simulink model "cdnlink_lb_wide_15a"  (Simulink 8.5)
settings: Solver=ode45  StartTime=0.0  StopTime=10.0  RelTol=1e-3
undefined symbols (not defined in the file): des, gcbh
(part 1 of 3)
settings Model: Creator=erwin2h  LastModifiedBy=erwin2h
settings DataIOCC: SignalLoggingSaveFormat=Dataset
settings OptimizationCC: ExpressionDepthLimit=128
settings DebuggingCC: UnderspecifiedInitializationDetection=Simplified  MergeDetectMultiDrivingBlocksExec=error  FcnCallInpInsideContextMsg=EnableAllAsError  StateNameClashWarn=none
settings GRTTargetCC: CombineOutputUpdateFcns=on  GRTInterface=off

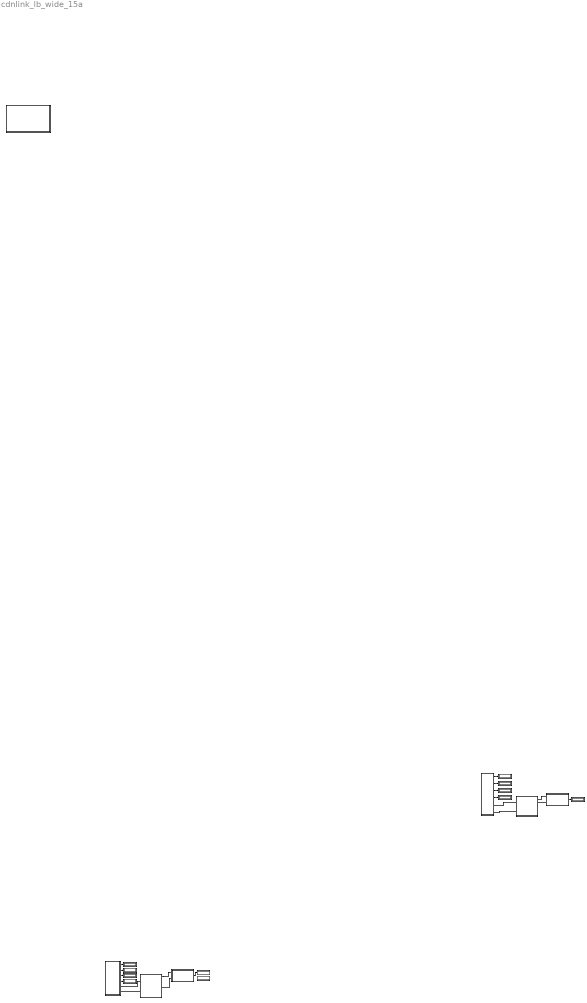
== system cdnlink_lb_wide_15a ==
  note: CDNLink
  note: Load Balancing Simulator
  note: Erwin Harahap
      | (R) 2015. Hiroaki Nishi Laboratory
      | Keio University, Yokohama.
      | Japan
  note: Last update: Sept 2015
  note: Fukuoka
  note: 1
  note: Kurashiki
  note: 3
  C1 : Subsystem
      mask Display: disp('Client 1');
  C3 : Subsystem
      mask Display: disp('Client\nv.2.0');
  Display{1..5,53,83..86,89} (11 alike) : Display
  Instrumentation : Subsystem
      mask Display: disp('Instrumentation')
  R1 : Subsystem
      mask Display: disp('Router 1');
  R3 : Subsystem
  S1 : Subsystem
      mask Display: disp('Surrogate Server 1');
  S3 : Subsystem
      mask Display: disp('Surrogate Server 1');
  wires:
  C1/1(Req sent) -> Display83/1
  C1/2(DNS sent) -> Display84/1
  C1/3(Req drop) -> Display85/1
  C1/4(DNS drop) -> Display86/1
  S1/1(Out1) -> Display89/1
  ? -> Display53/1
  C3/1(Req sent) -> Display1/1
  C3/2(DNS sent) -> Display2/1
  C3/3(Req drop) -> Display3/1
  C3/4(DNS drop) -> Display4/1
  S3/1(Out1) -> Display5/1
  connections:
  R1/RConn1 -- S1/LConn1
  S1/LConn2 -- R1/RConn5
  R1/LConn2 -- C1/RConn2
  R1/LConn1 -- C1/RConn1
  R3/LConn1 -- C3/RConn1
  R3/LConn2 -- C3/RConn2
  S3/LConn1 -- R3/RConn1
  S3/LConn2 -- R3/RConn2

== system cdnlink_lb_wide_15a/C1 ==
  note: CDNLink
  note: Client 1
  note: Erwin Harahap
      | (c) 2015. Hiroaki Nishi Laboratory
      | Keio University
      | Japan
  note: Ver. 2.0
  Packet Request Generator : Subsystem
      mask Display: disp('Packet \nGenerator')
  Processing Module1 : Subsystem
      mask Display: disp('Processing\nModule')
  Sink : Subsystem
      mask Display: disp('Sink')
  to router : PMIOPort  Port=1  Side=Right
  from Router : PMIOPort  Port=2  Side=Right
  Req sent : Outport
  DNS sent : Outport  Port=2
  Req drop : Outport  Port=3
  DNS drop : Outport  Port=4
  wires:
  Packet Request Generator/1(Out1) -> Req sent/1
  Packet Request Generator/2(Out2) -> DNS sent/1
  Sink/1(Out1) -> Req drop/1
  Sink/2(Out2) -> DNS drop/1
  connections:
  Processing Module1/LConn1 -- Packet Request Generator/RConn1
  Processing Module1/LConn2 -- from Router/RConn1
  Processing Module1/RConn1 -- to router/RConn1
  Processing Module1/RConn2 -- Sink/LConn1

== system cdnlink_lb_wide_15a/C3 ==
  note: Standard:
      | Arrival rate : 20 pkt/second = 1/20 = 0.05 sec/packet
      | Client service rate = 5 Mbps = 5*10^6 bps = 5*10^3/12 = 0.42*10^3 = 420 packet/second = 0.0024 s/packet = 2.4 ms/packet
      | Server service rate 10 Mbps = 10*10^6 bps = 10*10^3/12 = 0.83*10^3 = 830 packet/second = 0.0012 s/packet
      | SoR service rate : 10 Mbps
      | One packet size : 1500 bytes = 12000bps
      | 1 ms/packet = 1008 packet/s
  note: CDNLink
  note: Client 3
  Packet Request Generator : Subsystem
      mask Display: disp('Packet Generator\nv.1.02')
  Processing Module1 : Subsystem
      mask Display: disp('Client Processing Module\nv.1.03')
  Sink1 : Subsystem
      mask Display: disp('Sink')
  from Router : PMIOPort  Port=1  Side=Right
  to router : PMIOPort  Port=2  Side=Right
  Req sent : Outport
  DNS sent : Outport  Port=2
  Req drop : Outport  Port=3
  DNS drop : Outport  Port=4
  wires:
  Packet Request Generator/1(Out1) -> Req sent/1
  Packet Request Generator/2(Out2) -> DNS sent/1
  Sink1/1(Out1) -> Req drop/1
  Sink1/2(Out2) -> DNS drop/1
  connections:
  Processing Module1/LConn1 -- Packet Request Generator/RConn1
  Processing Module1/LConn2 -- from Router/RConn1
  Processing Module1/RConn1 -- to router/RConn1
  Sink1/LConn1 -- Processing Module1/RConn2

== system cdnlink_lb_wide_15a/Instrumentation ==
  note: CDNLink
  note: Instrumentation & Packet Monitoring
  note: v.1.0

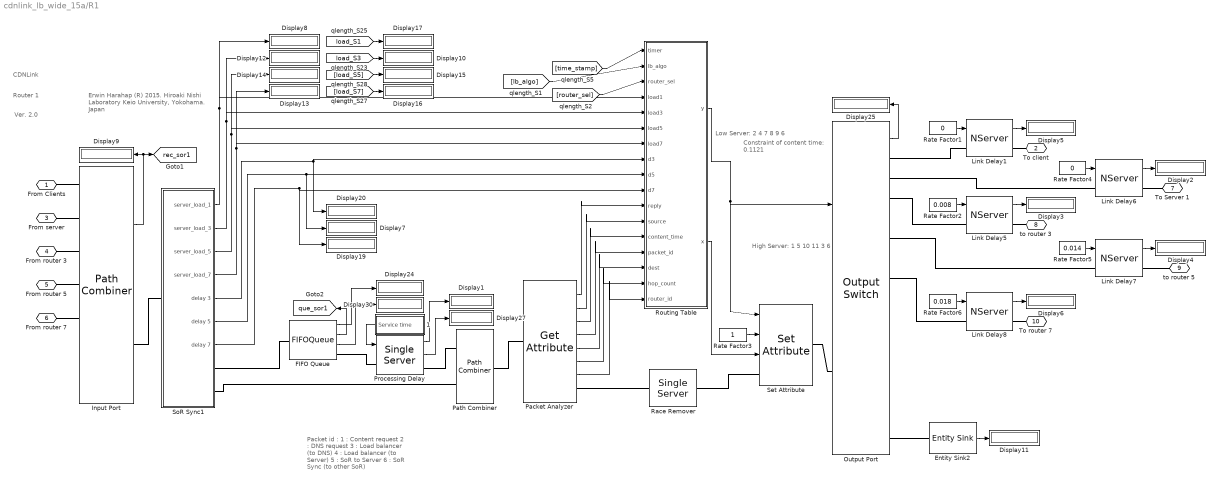
== system cdnlink_lb_wide_15a/R1 ==
  note: CDNLink
  note: Router 1
  note: High Server:
      | 1
      | 5
      | 10
      | 11
      | 3
      | 6
  note: Packet id :
      | 1 : Content request
      | 2 : DNS request
      | 3 : Load balancer (to DNS)
      | 4 : Load balancer (to Server)
      | 5 : SoR to Server
      | 6 : SoR Sync (to other SoR)
  note: Constraint of content time:
      | 0.1121
  note: Erwin Harahap
      | (R) 2015. Hiroaki Nishi Laboratory
      | Keio University, Yokohama.
      | Japan
  note: Low Server:
      | 2
      | 4
      | 7
      | 8
      | 9
      | 6
  note: Ver. 2.0
  " 1" : Subsystem
      mask Display: disp('M/M/1 Gen');
  Display{1..17,19..20,24..25,27,30} (23 alike) : Display
  Entity Sink2 : EntitySink  StatNumberArrived=on
  FIFO Queue : FIFOQueue  Capacity=2000  StatNumberDeparted=on  StatNumberInBlock=on  StatAverageQueueLength=on
      settings: OutputPortMap=o0,o1,o3
  Input Port : PathCombiner  NumberInputPorts=7  StatNumberDeparted=on
  Link Delay{1,5..8} (5 alike) : NServer  NumberOfServers=10000  ServiceTimeFrom=Signal port t  ServiceTime=0  StatNumberDeparted=on
  Output Port : OutputSwitch  NumberOutputPorts=15  SwitchingCriterion=From signal port p  AttributeName=cluster  StatNumberDeparted=on
  Packet Analyzer : GetAttribute  AttributeName=reply|source|content_time|packet_id|dest|hop_count|router_id  AttributeMissing=Error|Error|Error|Error|Error|Error|Error  AttributeDefaultValue=1|1|1|1|1|1|1  AttributeTreatAsVector=1|1|1|1|1|1|1  AttributeSendTiming=After entity departure|After entity departure|After entity departure|After entity departure|After entity departure|After entity departure|After entity departure  EvaluatedDefaultAttributeValue={ [];[];[];[];[];[];[]}
      settings: OutputPortMap=o1,o2,o3,o4,o5,o6,o7
  Path Combiner : PathCombiner  NumberInputPorts=2
  Processing Delay : SingleServer  ServiceTimeFrom=Signal port t  ServiceTime=0.000024  AttributeName=ServiceTimeRDC1  StatNumberDeparted=on  StatUtilization=on
      settings: OutputPortMap=o0,o5
  Race Remover : SingleServer  ServiceTime=0  AttributeName=ServiceTimeDNS
  Rate Factor1 : Constant  Value=0
  Rate Factor2 : Constant  Value=0.008
  Rate Factor3 : Constant
  Rate Factor4 : Constant  Value=0
  Rate Factor5 : Constant  Value=0.014
  Rate Factor6 : Constant  Value=0.018
  Routing Table : MATLAB Function  TreatAsAtomicUnit=on
  Set Attribute : SetAttribute  AttributeName=y_out|router_id|hop_count  AttributeFrom=Signal port|Signal port|Signal port  AttributeValue=2|1|1  AttributeTreatAsVector=1|1|1  EvaluatedAttributeValue={ [];[];[]}
      settings: InputPortMap=u0,u1,u2
  SoR Sync1 : Subsystem
  From Clients : PMIOPort  Port=1  Side=Left
  To client : PMIOPort  Port=2  Side=Left
  From server : PMIOPort  Port=3  Side=Right
  From router 3 : PMIOPort  Port=4  Side=Right
  From router 5 : PMIOPort  Port=5  Side=Right
  From router 7 : PMIOPort  Port=6  Side=Right
  To Server 1 : PMIOPort  Port=7  Side=Right
  to router 3 : PMIOPort  Port=8  Side=Right
  to router 5 : PMIOPort  Port=9  Side=Right
  To router 7 : PMIOPort  Port=10  Side=Right
  tag scope: que_sor1=global, rec_sor1=global
  wires:
  Output Port/1 -> Display25/1
  Packet Analyzer/1 -> Routing Table/11(reply)
  Packet Analyzer/2 -> Routing Table/12(source)
  Packet Analyzer/3 -> Routing Table/13(content_time)
  Packet Analyzer/4 -> Routing Table/14(packet_id)
  Packet Analyzer/5 -> Routing Table/15(dest)
  Input Port/1 -> [rec_sor1], Display9/1
  Entity Sink2/1 -> Display11/1
  Routing Table/1(y) -> Set Attribute/1, Output Port/1
  Rate Factor3/1 -> Set Attribute/2
  FIFO Queue/3 -> Display30/1
  Packet Analyzer/6 -> Routing Table/16(hop_count)
  Routing Table/2(x) -> Set Attribute/3
  SoR Sync1/2(server_load_3) -> Display12/1, Routing Table/5(load3)
  SoR Sync1/3(server_load_5) -> Display14/1, Routing Table/6(load5)
  SoR Sync1/4(server_load_7) -> Display13/1, Routing Table/7(load7)
  SoR Sync1/1(server_load_1) -> Display8/1, Routing Table/4(load1)
  [load_S3] -> Display10/1
  [load_S5] -> Display15/1
  [load_S7] -> Display16/1
  [load_S1] -> Display17/1
  FIFO Queue/1 -> Display24/1
  [time_stamp] -> Routing Table/1(timer)
  Packet Analyzer/7 -> Routing Table/17(router_id)
  FIFO Queue/2 -> [que_sor1]
  Processing Delay/2 -> Display27/1
  Processing Delay/1 -> Display1/1
  Rate Factor1/1 -> Link Delay1/1
  Rate Factor2/1 -> Link Delay5/1
  Rate Factor4/1 -> Link Delay6/1
  Rate Factor5/1 -> Link Delay7/1
  Rate Factor6/1 -> Link Delay8/1
  " 1"/1(Service time) -> Processing Delay/1
  [lb_algo] -> Routing Table/2(lb_algo)
  [router_sel] -> Routing Table/3(router_sel)
  Link Delay1/1 -> Display5/1
  Link Delay6/1 -> Display2/1
  Link Delay5/1 -> Display3/1
  Link Delay7/1 -> Display4/1
  Link Delay8/1 -> Display6/1
  SoR Sync1/5(delay 3) -> Display20/1, Routing Table/8(d3)
  SoR Sync1/6(delay 5) -> Routing Table/9(d5), Display7/1
  SoR Sync1/7(delay 7) -> Routing Table/10(d7), Display19/1
  connections:
  From Clients/RConn1 -- Input Port/LConn1
  From server/RConn1 -- Input Port/LConn2
  Packet Analyzer/RConn1 -- Race Remover/LConn1
  Processing Delay/RConn1 -- Path Combiner/LConn1
  Output Port/RConn1 -- Link Delay1/LConn1
  Link Delay6/LConn1 -- Output Port/RConn2
  Entity Sink2/LConn1 -- Output Port/RConn15
  Race Remover/RConn1 -- Set Attribute/LConn1
  Set Attribute/RConn1 -- Output Port/LConn1
  Input Port/RConn1 -- SoR Sync1/LConn1
  Path Combiner/RConn1 -- Packet Analyzer/LConn1
  SoR Sync1/RConn2 -- Path Combiner/LConn2
  SoR Sync1/RConn1 -- FIFO Queue/LConn1
  From router 3/RConn1 -- Input Port/LConn3
  From router 5/RConn1 -- Input Port/LConn4
  From router 7/RConn1 -- Input Port/LConn5
  FIFO Queue/RConn1 -- Processing Delay/LConn1
  Link Delay1/RConn1 -- To client/RConn1
  Link Delay6/RConn1 -- To Server 1/RConn1
  Link Delay5/RConn1 -- to router 3/RConn1
  Link Delay5/LConn1 -- Output Port/RConn3
  Link Delay7/RConn1 -- to router 5/RConn1
  Output Port/RConn5 -- Link Delay7/LConn1
  Link Delay8/RConn1 -- To router 7/RConn1
  Link Delay8/LConn1 -- Output Port/RConn7

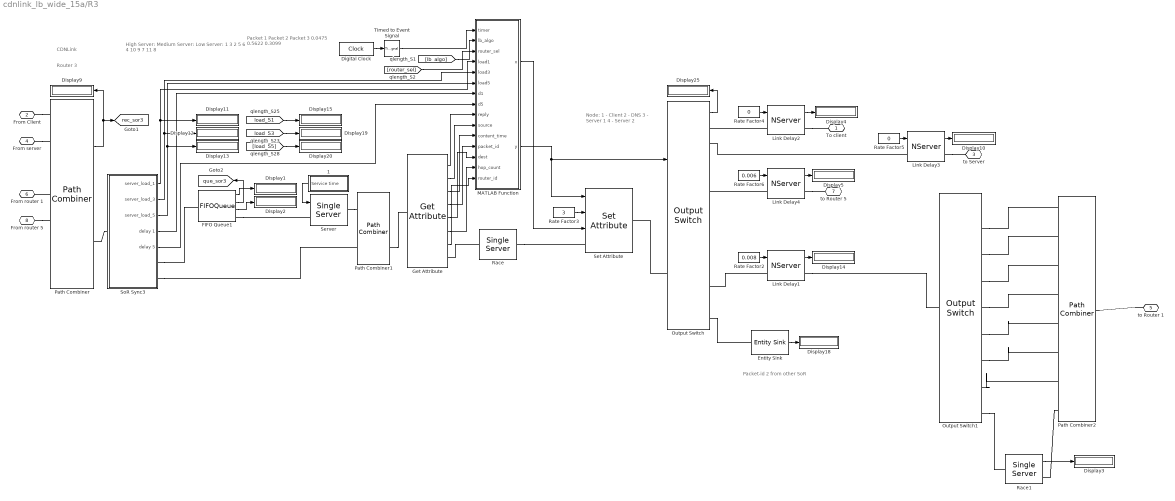
== system cdnlink_lb_wide_15a/R3 ==
  note: CDNLink
  note: Router 3
  note: Node:
      | 1 - Client
      | 2 - DNS
      | 3 - Server 1
      | 4 - Server 2
  note: High Server:    Medium Server:   Low Server:
      | 1                     3                          2
      | 5                     6                          4
      | 10                   9                          7
      | 11                                               8
  note: Packet 1    Packet 2   Packet 3
      | 0.0475      0.5622      0.3099
  note: Packet-id 2 from other SoR
  " 1" : Subsystem
      mask Display: disp('M/M/1 Gen');
  Digital Clock : DigitalClock
  Display{1..5,9..15,18..20,25} (16 alike) : Display
  Entity Sink : EntitySink  StatNumberArrived=on
  FIFO Queue1 : FIFOQueue  Capacity=2000  StatNumberDeparted=on  StatNumberInBlock=on  StatAverageQueueLength=on
      settings: OutputPortMap=o0,o1,o3
  Get Attribute : GetAttribute  AttributeName=reply|source|content_time|packet_id|dest|hop_count|router_id  AttributeMissing=Error|Error|Error|Error|Error|Error|Default value  AttributeDefaultValue=1|1|1|1|1|1|0  AttributeTreatAsVector=1|1|1|1|1|1|1  AttributeSendTiming=After entity departure|After entity departure|After entity departure|After entity departure|After entity departure|After entity departure|After entity departure  EvaluatedDefaultAttributeValue={ [];[];[];[];[];[];0}
      settings: OutputPortMap=o1,o2,o3,o4,o5,o6,o7
  Link Delay{1..4} (4 alike) : NServer  NumberOfServers=10000  ServiceTimeFrom=Signal port t  ServiceTime=0  StatNumberDeparted=on
  MATLAB Function : MATLAB Function  TreatAsAtomicUnit=on
  Output Switch : OutputSwitch  NumberOutputPorts=13  SwitchingCriterion=From signal port p  AttributeName=cluster  StatNumberDeparted=on
  Output Switch1 : OutputSwitch  NumberOutputPorts=8  SwitchingCriterion=From attribute  AttributeName=packet_id  StatNumberDeparted=on
  Path Combiner : PathCombiner  NumberInputPorts=7  StatNumberDeparted=on
  Path Combiner1 : PathCombiner  NumberInputPorts=2  StatNumberDeparted=on
  Path Combiner2 : PathCombiner  NumberInputPorts=8
  Race : SingleServer  ServiceTime=0  AttributeName=ServiceTimeDNS
  Race1 : SingleServer  ServiceTime=0  AttributeName=ServiceTimeDNS  StatNumberDeparted=on
  Rate Factor2 : Constant  Value=0.008
  Rate Factor3 : Constant  Value=3
  Rate Factor4 : Constant  Value=0
  Rate Factor5 : Constant  Value=0
  Rate Factor6 : Constant  Value=0.006
  Server : SingleServer  ServiceTimeFrom=Signal port t  ServiceTime=0.0006  AttributeName=ServiceTimeRDC1
  Set Attribute : SetAttribute  AttributeName=y_out|router_id|hop_count  AttributeFrom=Signal port|Signal port|Signal port  AttributeValue=2|1|1  AttributeTreatAsVector=1|1|1  EvaluatedAttributeValue={ [];[];[]}
      settings: InputPortMap=u0,u1,u2
  SoR Sync3 : Subsystem
  Timed to Event Signal : TimedToEventSignal
  To client : PMIOPort  Port=1  Side=Left
  From Client : PMIOPort  Port=2  Side=Left
  to Server : PMIOPort  Port=3  Side=Right
  From server : PMIOPort  Port=4  Side=Right
  to Router 1 : PMIOPort  Port=5  Side=Right
  From router 1 : PMIOPort  Port=6  Side=Right
  to Router 5 : PMIOPort  Port=7  Side=Right
  From router 5 : PMIOPort  Port=8  Side=Right
  tag scope: que_sor3=global, rec_sor3=global
  wires:
  Path Combiner/1 -> [rec_sor3], Display9/1
  MATLAB Function/2(y) -> Set Attribute/1, Output Switch/1
  Output Switch/1 -> Display25/1
  Link Delay2/1 -> Display4/1
  Link Delay4/1 -> Display5/1
  Link Delay3/1 -> Display10/1
  Link Delay1/1 -> Display14/1
  " 1"/1(Service time) -> Server/1
  Get Attribute/1 -> MATLAB Function/9(reply)
  Get Attribute/2 -> MATLAB Function/10(source)
  Get Attribute/3 -> MATLAB Function/11(content_time)
  Get Attribute/4 -> MATLAB Function/12(packet_id)
  Get Attribute/5 -> MATLAB Function/13(dest)
  Entity Sink/1 -> Display18/1
  Rate Factor3/1 -> Set Attribute/2
  Get Attribute/6 -> MATLAB Function/14(hop_count)
  MATLAB Function/1(x) -> Set Attribute/3
  SoR Sync3/1(server_load_1) -> Display11/1, MATLAB Function/4(load1)
  SoR Sync3/3(server_load_5) -> Display13/1, MATLAB Function/6(load5)
  [load_S1] -> Display15/1
  [load_S3] -> Display19/1
  [load_S5] -> Display20/1
  SoR Sync3/2(server_load_3) -> Display12/1, MATLAB Function/5(load3)
  Digital Clock/1 -> Timed to Event Signal/1
  Timed to Event Signal/1 -> MATLAB Function/1(timer)
  Get Attribute/7 -> MATLAB Function/15(router_id)
  FIFO Queue1/2 -> [que_sor3]
  Rate Factor2/1 -> Link Delay1/1
  Rate Factor4/1 -> Link Delay2/1
  Rate Factor5/1 -> Link Delay3/1
  Rate Factor6/1 -> Link Delay4/1
  FIFO Queue1/3 -> Display2/1
  FIFO Queue1/1 -> Display1/1
  [lb_algo] -> MATLAB Function/2(lb_algo)
  [router_sel] -> MATLAB Function/3(router_sel)
  Race1/1 -> Display3/1
  SoR Sync3/4(delay 1) -> MATLAB Function/7(d1)
  SoR Sync3/5(delay 5) -> MATLAB Function/8(d5)
  connections:
  SoR Sync3/RConn1 -- FIFO Queue1/LConn1
  From Client/RConn1 -- Path Combiner/LConn1
  From server/RConn1 -- Path Combiner/LConn2
  Get Attribute/RConn1 -- Race/LConn1
  Link Delay2/RConn1 -- To client/RConn1
  Link Delay4/RConn1 -- to Router 5/RConn1
  Link Delay2/LConn1 -- Output Switch/RConn1
  Link Delay3/LConn1 -- Output Switch/RConn2
  Path Combiner/LConn4 -- From router 1/RConn1
  Link Delay1/RConn1 -- Output Switch1/LConn1
  From router 5/RConn1 -- Path Combiner/LConn5
  Link Delay3/RConn1 -- to Server/RConn1
  Output Switch/RConn13 -- Entity Sink/LConn1
  Link Delay1/LConn1 -- Output Switch/RConn11
  Link Delay4/LConn1 -- Output Switch/RConn5
  Race/RConn1 -- Set Attribute/LConn1
  Output Switch/LConn1 -- Set Attribute/RConn1
  Path Combiner/RConn1 -- SoR Sync3/LConn1
  Server/RConn1 -- Path Combiner1/LConn1
  Path Combiner1/RConn1 -- Get Attribute/LConn1
  SoR Sync3/RConn2 -- Path Combiner1/LConn2
  FIFO Queue1/RConn1 -- Server/LConn1
  to Router 1/RConn1 -- Path Combiner2/RConn1
  Output Switch1/RConn1 -- Path Combiner2/LConn1
  Output Switch1/RConn2 -- Path Combiner2/LConn2
  Output Switch1/RConn3 -- Path Combiner2/LConn3
  Output Switch1/RConn4 -- Path Combiner2/LConn4
  Output Switch1/RConn5 -- Path Combiner2/LConn5
  Output Switch1/RConn6 -- Path Combiner2/LConn6
  Output Switch1/RConn7 -- Path Combiner2/LConn7
  Output Switch1/RConn8 -- Race1/LConn1
  Race1/RConn1 -- Path Combiner2/LConn8

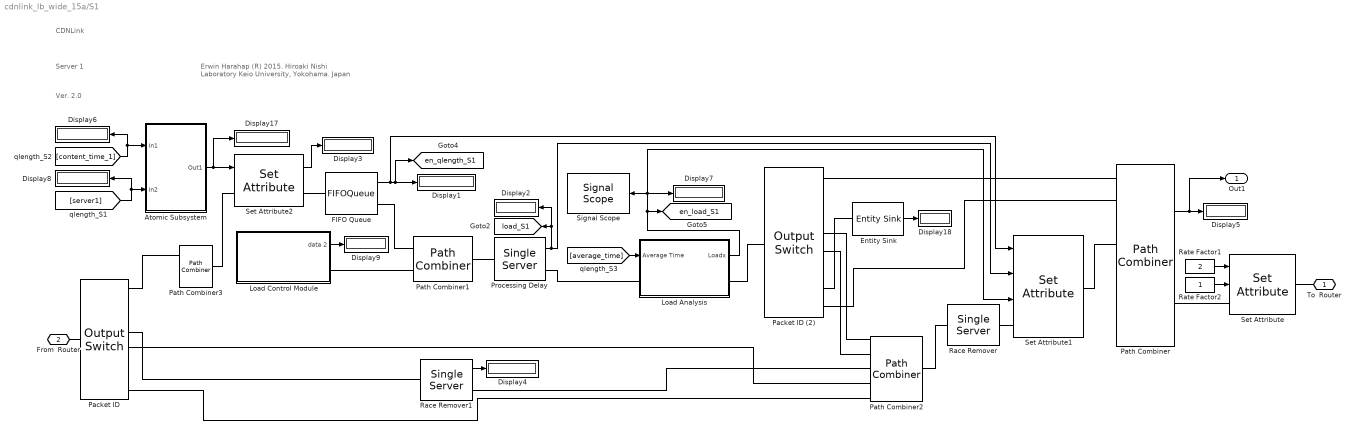
== system cdnlink_lb_wide_15a/S1 ==
  note: CDNLink
  note: Server 1
  note: Erwin Harahap
      | (R) 2015. Hiroaki Nishi Laboratory
      | Keio University, Yokohama.
      | Japan
  note: Ver. 2.0
  Atomic Subsystem : Subsystem  TreatAsAtomicUnit=on
  Display{1..9,17..18} (11 alike) : Display
  Entity Sink : EntitySink  StatNumberArrived=on
  FIFO Queue : FIFOQueue  Capacity=2000  StatNumberInBlock=on
      settings: OutputPortMap=o1
  Load Analysis : Subsystem
      mask Display: disp('Load Analysis');
  Load Control Module : Subsystem
      mask Display: disp('Load Control Module');
  Packet ID : OutputSwitch  NumberOutputPorts=8  SwitchingCriterion=From attribute  AttributeName=packet_id
  Packet ID (2) : OutputSwitch  NumberOutputPorts=8  SwitchingCriterion=From attribute  AttributeName=packet_id
  Path Combiner : PathCombiner  NumberInputPorts=8  StatNumberDeparted=on
  Path Combiner1 : PathCombiner  NumberInputPorts=2
  Path Combiner2 : PathCombiner  NumberInputPorts=5
  Path Combiner3 : PathCombiner  NumberInputPorts=2
  Processing Delay : SingleServer  ServiceTimeFrom=Attribute  ServiceTime=0.0006  AttributeName=content_time  StatUtilization=on
      settings: OutputPortMap=o5
  Race Remover : SingleServer  ServiceTime=0  AttributeName=ServiceTimeDNS
  Race Remover1 : SingleServer  ServiceTime=0  AttributeName=ServiceTimeDNS  StatNumberDeparted=on
  Rate Factor1 : Constant  Value=2
  Rate Factor2 : Constant
  Set Attribute : SetAttribute  AttributeName=reply|last_server  AttributeFrom=Signal port|Signal port  AttributeValue=2|1  AttributeTreatAsVector=1|1  EvaluatedAttributeValue={ [];[]}
      settings: InputPortMap=u0,u1
  Set Attribute1 : SetAttribute  AttributeName=qlength1|av_load1|en_load1  AttributeFrom=Signal port|Signal port|Signal port  AttributeValue=1|1|1  AttributeTreatAsVector=1|1|1  EvaluatedAttributeValue={ [];[];[]}
      settings: InputPortMap=u0,u1,u2
  Set Attribute2 : SetAttribute  AttributeName=content_time  AttributeFrom=Signal port  StatNumberDeparted=on  EvaluatedAttributeValue={ []}
  Signal Scope : SignalScope  LoadFcn=des.scope.CallbackSupport('seLoadFcn',gcbh)  StartFcn=des.scope.CallbackSupport('seStartFcn',gcbh)  StopFcn=des.scope.CallbackSupport('seStopFcn',gcbh)  PlotType=Continuous  OpenScopeAtSimStart=off  XMax=250  DataStoreOption=Unlimited
      settings: CopyFcn=des.scope.CallbackSupport('seCopyFcn',gcbh)  DeleteFcn=des.scope.CallbackSupport('seDeleteFcn',gcbh)  PreSaveFcn=des.scope.CallbackSupport('sePreSaveFcn',gcbh)  NameChangeFcn=des.scope.CallbackSupport('seNameChangeFcn',gcbh)  OpenFcn=des.scope.CallbackSupport('seOpenFcn',gcbh)  YMax=1
  To  Router : PMIOPort  Port=1  Side=Left
  From  Router : PMIOPort  Port=2  Side=Left
  Out1 : Outport
  tag scope: en_load_S1=global, en_qlength_S1=global, load_S1=global
  wires:
  [server1] -> Display8/1, Atomic Subsystem/2(In2)
  Atomic Subsystem/1(Out1) -> Set Attribute2/1, Display17/1
  Set Attribute2/1 -> Display3/1
  Path Combiner/1 -> Out1/1, Display5/1
  Rate Factor1/1 -> Set Attribute/1
  Rate Factor2/1 -> Set Attribute/2
  Entity Sink/1 -> Display18/1
  Load Control Module/1(data 2) -> Display9/1
  [content_time_1] -> Display6/1, Atomic Subsystem/1(In1)
  Processing Delay/1 -> Display2/1, [load_S1], Set Attribute1/2
  FIFO Queue/1 -> Set Attribute1/1, [en_qlength_S1], Display1/1
  Load Analysis/1(Loadx) -> Set Attribute1/3, Display7/1, Signal Scope/1, [en_load_S1]
  [average_time] -> Load Analysis/1(Average Time)
  Race Remover1/1 -> Display4/1
  connections:
  Set Attribute1/RConn1 -- Path Combiner/LConn4
  Set Attribute2/RConn1 -- FIFO Queue/LConn1
  From  Router/RConn1 -- Packet ID/LConn1
  FIFO Queue/RConn1 -- Path Combiner1/LConn1
  Path Combiner/RConn1 -- Set Attribute/LConn1
  Path Combiner1/RConn1 -- Processing Delay/LConn1
  Path Combiner2/LConn4 -- Packet ID/RConn5
  Packet ID/RConn4 -- Race Remover1/LConn1
  Processing Delay/RConn1 -- Load Analysis/LConn1
  Packet ID (2)/RConn1 -- Path Combiner/LConn1
  Path Combiner2/RConn1 -- Race Remover/LConn1
  Packet ID (2)/RConn4 -- Path Combiner2/LConn1
  Packet ID (2)/RConn5 -- Path Combiner2/LConn2
  Race Remover/RConn1 -- Set Attribute1/LConn1
  Packet ID (2)/RConn7 -- Entity Sink/LConn1
  To  Router/RConn1 -- Set Attribute/RConn1
  Load Control Module/RConn1 -- Path Combiner1/LConn2
  Load Analysis/RConn1 -- Packet ID (2)/LConn1
  Race Remover1/RConn1 -- Path Combiner2/LConn3
  Set Attribute2/LConn1 -- Path Combiner3/RConn1
  Packet ID/RConn1 -- Path Combiner3/LConn1
  Packet ID/RConn8 -- Path Combiner2/LConn5
  Packet ID (2)/RConn8 -- Path Combiner/LConn2

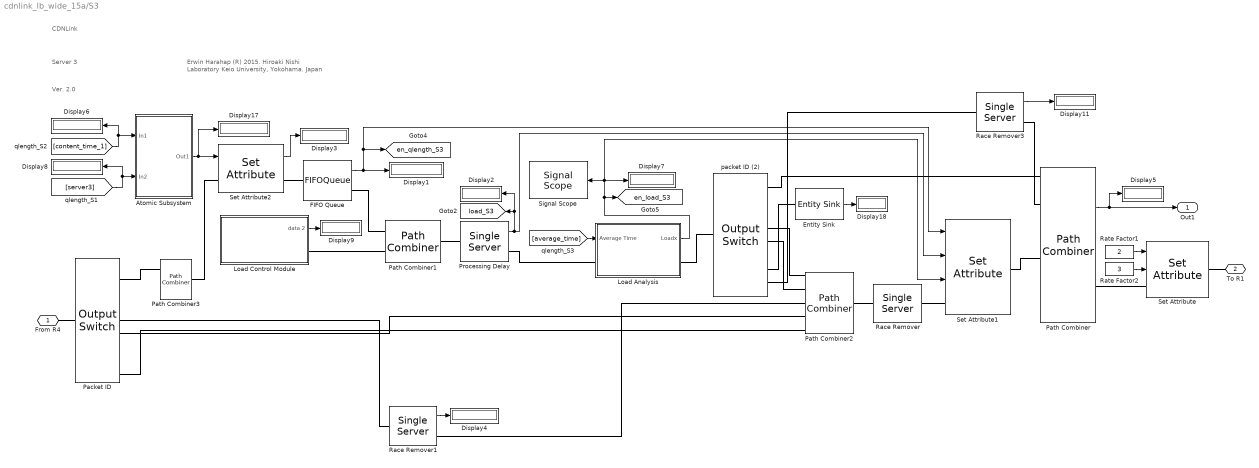
== system cdnlink_lb_wide_15a/S3 ==
  note: CDNLink
  note: Server 3
  note: Erwin Harahap
      | (R) 2015. Hiroaki Nishi Laboratory
      | Keio University, Yokohama.
      | Japan
  note: Ver. 2.0
  Atomic Subsystem : Subsystem  TreatAsAtomicUnit=on
  Display{1..9,11,17..18} (12 alike) : Display
  Entity Sink : EntitySink  StatNumberArrived=on
  FIFO Queue : FIFOQueue  Capacity=2000  StatNumberInBlock=on
      settings: OutputPortMap=o1
  Load Analysis : Subsystem
      mask Display: disp('Load Analysis');
  Load Control Module : Subsystem
      mask Display: disp('Load Control Module');
  Packet ID : OutputSwitch  NumberOutputPorts=8  SwitchingCriterion=From attribute  AttributeName=packet_id  StatNumberDeparted=on
  Path Combiner : PathCombiner  NumberInputPorts=6  StatNumberDeparted=on
  Path Combiner1 : PathCombiner  NumberInputPorts=2
  Path Combiner2 : PathCombiner  NumberInputPorts=5
  Path Combiner3 : PathCombiner  NumberInputPorts=2
  Processing Delay : SingleServer  ServiceTimeFrom=Attribute  ServiceTime=0.0006  AttributeName=content_time  StatUtilization=on
      settings: OutputPortMap=o5
  Race Remover : SingleServer  ServiceTime=0  AttributeName=ServiceTimeDNS
  Race Remover1 : SingleServer  ServiceTime=0  AttributeName=ServiceTimeDNS  StatNumberDeparted=on
  Race Remover3 : SingleServer  ServiceTime=0  AttributeName=ServiceTimeDNS  StatNumberDeparted=on
  Rate Factor1 : Constant  Value=2
  Rate Factor2 : Constant  Value=3
  Set Attribute : SetAttribute  AttributeName=reply|last_server  AttributeFrom=Signal port|Signal port  AttributeValue=2|1  AttributeTreatAsVector=1|1  EvaluatedAttributeValue={ [];[]}
      settings: InputPortMap=u0,u1
  Set Attribute1 : SetAttribute  AttributeName=qlength3|av_load3|en_load3  AttributeFrom=Signal port|Signal port|Signal port  AttributeValue=1|1|1  AttributeTreatAsVector=1|1|1  EvaluatedAttributeValue={ [];[];[]}
      settings: InputPortMap=u0,u1,u2
  Set Attribute2 : SetAttribute  AttributeName=content_time  AttributeFrom=Signal port  StatNumberDeparted=on  EvaluatedAttributeValue={ []}
  Signal Scope : SignalScope  LoadFcn=des.scope.CallbackSupport('seLoadFcn',gcbh)  StartFcn=des.scope.CallbackSupport('seStartFcn',gcbh)  StopFcn=des.scope.CallbackSupport('seStopFcn',gcbh)  PlotType=Continuous  OpenScopeAtSimStart=off  XMax=250  DataStoreOption=Unlimited
      settings: CopyFcn=des.scope.CallbackSupport('seCopyFcn',gcbh)  DeleteFcn=des.scope.CallbackSupport('seDeleteFcn',gcbh)  PreSaveFcn=des.scope.CallbackSupport('sePreSaveFcn',gcbh)  NameChangeFcn=des.scope.CallbackSupport('seNameChangeFcn',gcbh)  OpenFcn=des.scope.CallbackSupport('seOpenFcn',gcbh)  YMax=1
  packet ID (2) : OutputSwitch  NumberOutputPorts=8  SwitchingCriterion=From attribute  AttributeName=packet_id
  From R4 : PMIOPort  Port=1  Side=Left
  To R1 : PMIOPort  Port=2  Side=Left
  Out1 : Outport
  tag scope: en_load_S3=global, en_qlength_S3=global, load_S3=global
  wires:
  [server3] -> Display8/1, Atomic Subsystem/2(In2)
  Atomic Subsystem/1(Out1) -> Set Attribute2/1, Display17/1
  Set Attribute2/1 -> Display3/1
  Path Combiner/1 -> Display5/1, Out1/1
  Rate Factor1/1 -> Set Attribute/1
  Rate Factor2/1 -> Set Attribute/2
  Entity Sink/1 -> Display18/1
  Load Control Module/1(data 2) -> Display9/1
  [content_time_1] -> Display6/1, Atomic Subsystem/1(In1)
  Processing Delay/1 -> Display2/1, [load_S3], Set Attribute1/2
  FIFO Queue/1 -> [en_qlength_S3], Set Attribute1/1, Display1/1
  Load Analysis/1(Loadx) -> Set Attribute1/3, Display7/1, Signal Scope/1, [en_load_S3]
  [average_time] -> Load Analysis/1(Average Time)
  Race Remover1/1 -> Display4/1
  Race Remover3/1 -> Display11/1
  connections:
  Set Attribute1/RConn1 -- Path Combiner/LConn4
  Set Attribute2/RConn1 -- FIFO Queue/LConn1
  From R4/RConn1 -- Packet ID/LConn1
  FIFO Queue/RConn1 -- Path Combiner1/LConn1
  Path Combiner/RConn1 -- Set Attribute/LConn1
  Path Combiner1/RConn1 -- Processing Delay/LConn1
  Path Combiner2/LConn4 -- Packet ID/RConn5
  Packet ID/RConn4 -- Race Remover1/LConn1
  Processing Delay/RConn1 -- Load Analysis/LConn1
  packet ID (2)/RConn1 -- Path Combiner/LConn1
  Path Combiner2/RConn1 -- Race Remover/LConn1
  packet ID (2)/RConn4 -- Path Combiner2/LConn1
  packet ID (2)/RConn5 -- Path Combiner2/LConn2
  Race Remover/RConn1 -- Set Attribute1/LConn1
  packet ID (2)/RConn7 -- Entity Sink/LConn1
  To R1/RConn1 -- Set Attribute/RConn1
  Load Control Module/RConn1 -- Path Combiner1/LConn2
  Load Analysis/RConn1 -- packet ID (2)/LConn1
  Race Remover1/RConn1 -- Path Combiner2/LConn3
  Packet ID/RConn1 -- Path Combiner3/LConn1
  Path Combiner2/LConn5 -- Packet ID/RConn8
  Path Combiner3/RConn1 -- Set Attribute2/LConn1
  packet ID (2)/RConn8 -- Race Remover3/LConn1
  Race Remover3/RConn1 -- Path Combiner/LConn2

== system cdnlink_lb_wide_15a/C1/Packet Request Generator ==
  note: CDNLink
  note: Client Packet Generator - CLIENT 1
  note: Standard:
      | Arrival rate : 20 pkt/second = 1/20 = 0.05 sec/packet
      | Client service rate = 5 Mbps = 5*10^6 bps = 5*10^6/12000 = 5*10^3/12 = 0.42*10^3 = 420 packet/second = 0.0024 s/packet = 2.4 ms/packet
      | Server service rate 10 Mbps = 10*10^6 bps = 10*10^3/12 = 0.83*10^3 = 830 packet/second = 0.0012 s/packet
      | SoR service rate : 10 Mbps
      | One packet size : 1500 bytes = 12000bps
      | 1 ms/packet = 1008 packet/s
  note: Node:
      | 1 - Client                     4 - Load Balancer
      | 2 - DNS Server            5 - Router
      | 3 - Surrogate Server
  note: packet-id
      | 1 - Request packet
      | 2 - DNS packet
  note: packet-id:  1
      | Request packet
      | Seed: 185274
  note: packet-id: 2
      | DNS packet
  note: Uniform Distribution
      | 0 to 5 (in sec)
  note: M/M/1
      | Poisson Distribution
  note: v.1.03
  note: Source:
      | 1 - Cluster 1
      | 2 - Cluster 2
      | etc.
  note: Standard:
      | Arrival rate : 20 pkt/second = 1/20 = 0.05 sec/packet
      | Client service rate = 5 Mbps = 5*10^6 bps = 5*10^3/12 = 0.42*10^3 = 420 packet/second = 0.0024 s/packet = 2.4 ms/packet
      | Server service rate 10 Mbps = 10*10^6 bps = 10*10^3/12 = 0.83*10^3 = 830 packet/second = 0.0012 s/packet
      | SoR service rate : 10 Mbps
      | One packet size : 1500 bytes = 12000bps
      | 1 ms/packet = 1008 packet/s
  "  " : Subsystem  mask(Exponential Random Number Generator){seed=185274}
      mask prompts: seed "Initial seed"
      mask help: Output exponentially distributed random numbers with the input rate. Output is repeatable for a given seed.
      mask Display: disp('Exponential\n Distribution');
  DNS Req Generator : TimeBasedEntityGenerator  GenerateEntitiesUpon=Intergeneration time from port t  Distribution=Uniform  Period=10  InitialSeed=1715331  Maximum=5  Mean=0.05  ResponseWhenBlocked=Error  EntityType=Standard  StatNumberDeparted=on  StatAverageIntergenerationTime=on
      settings: OutputPortMap=o0,o2
  Display{1..4,6..7,11} (7 alike) : Display
  Packet  Generator : TimeBasedEntityGenerator  GenerateEntitiesUpon=Intergeneration time from port t  Distribution=Exponential  Period=0.05  InitialSeed=1234  Mean=0.05  GenerateEntityAtSimulationStart=off  EntityType=Standard  StatNumberDeparted=on
  Packet Config : Subsystem
      mask Display: disp('Packet Config')
  Path Combiner : PathCombiner  NumberInputPorts=2
  Rate Factor{1,5..8} (5 alike) : Constant
  Rate Factor10 : Constant  Value=0
  Rate Factor2 : Constant  Value=0
  Rate Factor3 : Constant  Value=2
  Rate Factor9 : Constant  Value=0
  Set Attribute1 : SetAttribute  AttributeName=node|reply|source|hop_count|router_id  AttributeFrom=Signal port|Signal port|Signal port|Signal port|Signal port  AttributeValue=1|1|1|1|1  AttributeTreatAsVector=1|1|1|1|1  EvaluatedAttributeValue={ [];[];[];[];[]}
      settings: InputPortMap=u0,u1,u2,u3,u4
  Set Attribute2 : SetAttribute  AttributeName=packet_id|content_time|dest  AttributeFrom=Signal port|Signal port|Signal port  AttributeValue=1|1|1  AttributeTreatAsVector=1|1|1  StatNumberDeparted=on  EvaluatedAttributeValue={ [];[];[]}
      settings: InputPortMap=u0,u1,u2
  Set Attribute6 : SetAttribute  AttributeName=packet_id  AttributeFrom=Signal port  StatNumberDeparted=on  EvaluatedAttributeValue={ []}
  Conn1 : PMIOPort  Port=1  Side=Right
  Out1 : Outport
  Out2 : Outport  Port=2
  wires:
  Rate Factor6/1 -> Set Attribute1/3
  Rate Factor7/1 -> Set Attribute1/2
  Rate Factor1/1 -> Set Attribute1/1
  Rate Factor3/1 -> Set Attribute2/1
  Rate Factor8/1 -> Set Attribute2/3
  Rate Factor2/1 -> Set Attribute2/2
  Set Attribute2/1 -> Out2/1, Display6/1
  [lambda_dns] -> DNS Req Generator/1, Display2/1
  Set Attribute6/1 -> Display1/1, Out1/1
  Rate Factor5/1 -> Set Attribute6/1
  DNS Req Generator/2 -> Display7/1
  DNS Req Generator/1 -> Display3/1
  [lambda1] -> "  "/1(Arrival Rate), Display4/1
  "  "/1(Out1) -> Packet  Generator/1
  Packet  Generator/1 -> Display11/1
  Rate Factor9/1 -> Set Attribute1/4
  Rate Factor10/1 -> Set Attribute1/5
  connections:
  Path Combiner/RConn1 -- Set Attribute1/LConn1
  Set Attribute6/RConn1 -- Path Combiner/LConn1
  Packet Config/RConn1 -- Set Attribute6/LConn1
  Packet  Generator/RConn1 -- Packet Config/LConn1
  Set Attribute2/RConn1 -- Path Combiner/LConn2
  Conn1/RConn1 -- Set Attribute1/RConn1
  DNS Req Generator/RConn1 -- Set Attribute2/LConn1

== system cdnlink_lb_wide_15a/C1/Processing Module1 ==
  note: CDNLink
  note: Client Processing Module
  note: packet-id
      | 1 - Request packet
      | 2 - DNS packet
  note: Destination obtained from
      | DNS packet
  note: v.1.0
  AvgDelay SQ{6..9} (4 alike) : Display
  Display5 : Display
  Get Attribute1 : GetAttribute  AttributeName=dest  AttributeMissing=Default value  StatNumberDeparted=on  EvaluatedDefaultAttributeValue={ 1}
      settings: OutputPortMap=o0,o1
  Packet Id : OutputSwitch  NumberOutputPorts=2  SwitchingCriterion=From attribute  InitialSeed=13927  AttributeName=packet_id  InitialConditionsOpt=on
  Packet_id : OutputSwitch  NumberOutputPorts=2  SwitchingCriterion=From attribute  AttributeName=packet_id
  Packet_id1 : OutputSwitch  NumberOutputPorts=2  SwitchingCriterion=From attribute  AttributeName=packet_id
  Path Combiner : PathCombiner  NumberInputPorts=2
  Path Combiner1 : PathCombiner  NumberInputPorts=2
  Path Combiner2 : PathCombiner  NumberInputPorts=2  StatNumberDeparted=on
  Set Attribute14 : SetAttribute  AttributeName=dest  AttributeFrom=Signal port  AttributeValue=2  StatNumberDeparted=on  EvaluatedAttributeValue={ []}
  Start Timer : StartTimer  StatNumberDeparted=on
  From  Packet Generator : PMIOPort  Port=1  Side=Left
  To Router : PMIOPort  Port=2  Side=Right
  to sink : PMIOPort  Port=3  Side=Right
  From Router : PMIOPort  Port=4  Side=Left
  tag scope: dest_C1=global
  wires:
  Get Attribute1/1 -> AvgDelay SQ8/1
  Set Attribute14/1 -> AvgDelay SQ6/1
  Start Timer/1 -> AvgDelay SQ9/1
  Get Attribute1/2 -> [dest_C1], Set Attribute14/1, AvgDelay SQ7/1
  Path Combiner2/1 -> Display5/1
  connections:
  Path Combiner1/RConn1 -- To Router/RConn1
  Path Combiner/RConn1 -- Packet Id/LConn1
  Start Timer/RConn1 -- Path Combiner1/LConn1
  From  Packet Generator/RConn1 -- Packet_id/LConn1
  Packet_id/RConn2 -- Path Combiner/LConn2
  Packet_id/RConn1 -- Set Attribute14/LConn1
  Packet Id/RConn1 -- Start Timer/LConn1
  Set Attribute14/RConn1 -- Path Combiner/LConn1
  From Router/RConn1 -- Packet_id1/LConn1
  Packet_id1/RConn2 -- Get Attribute1/LConn1
  Get Attribute1/RConn1 -- Path Combiner2/LConn2
  Packet_id1/RConn1 -- Path Combiner2/LConn1
  Path Combiner2/RConn1 -- to sink/RConn1
  Packet Id/RConn2 -- Path Combiner1/LConn2

== system cdnlink_lb_wide_15a/C1/Sink ==
  note: Packet ID
      | 1 : Client request & Data
      | 2 : DNS request
  note: Load 1
  note: Load 3
  note: Load 5
  note: Load 7
  Display{1..3,8,10,17,19..21,23..24,26..27} (13 alike) : Display
  Entity Sink : EntitySink  StatNumberArrived=on
  Entity Sink1 : EntitySink  StatNumberArrived=on
  "Output Switch: Packet ID " : OutputSwitch  NumberOutputPorts=2  SwitchingCriterion=From attribute  AttributeName=packet_id
  Packet Analyzer1 : GetAttribute  AttributeName=reply|source|content_time|packet_id|router_hop|last_server  AttributeMissing=Error|Error|Error|Error|Error|Error  AttributeDefaultValue=1|1|1|1|1|1  AttributeTreatAsVector=1|1|1|1|1|1  AttributeSendTiming=After entity departure|After entity departure|After entity departure|After entity departure|After entity departure|After entity departure  EvaluatedDefaultAttributeValue={ [];[];[];[];[];[]}
      settings: OutputPortMap=o1,o2,o3,o4,o5,o6
  Read Timer : ReadTimer  TimerModeOption=Ignore  StatNumberDeparted=on  StatTimeElapsed=on  StatAverageTimeElapsed=on
      settings: OutputPortMap=o0,o2,o3
  SoR RAND Server 1 : Scope
      settings: ShowLegends=on  TimeRange=250  YMin=0  YMax=175  SaveName=ScopeData13
  Conn1 : PMIOPort  Port=1  Side=Left
  Out1 : Outport
  Out2 : Outport  Port=2
  tag scope: rtt_avg_c1=global, rtt_elaps_c1=global
  wires:
  Entity Sink/1 -> Display8/1, Out1/1
  Read Timer/1 -> Display1/1
  Entity Sink1/1 -> Out2/1, Display2/1
  Read Timer/2 -> [rtt_elaps_c1]
  Read Timer/3 -> [rtt_avg_c1]
  Packet Analyzer1/1 -> Display10/1
  Packet Analyzer1/2 -> Display17/1
  Packet Analyzer1/3 -> Display19/1
  Packet Analyzer1/4 -> Display20/1
  Packet Analyzer1/5 -> SoR RAND Server 1/1, Display21/1
  Packet Analyzer1/6 -> Display3/1
  connections:
  Conn1/RConn1 -- "Output Switch: Packet ID "/LConn1
  "Output Switch: Packet ID "/RConn1 -- Read Timer/LConn1
  "Output Switch: Packet ID "/RConn2 -- Entity Sink1/LConn1
  Read Timer/RConn1 -- Entity Sink/LConn1

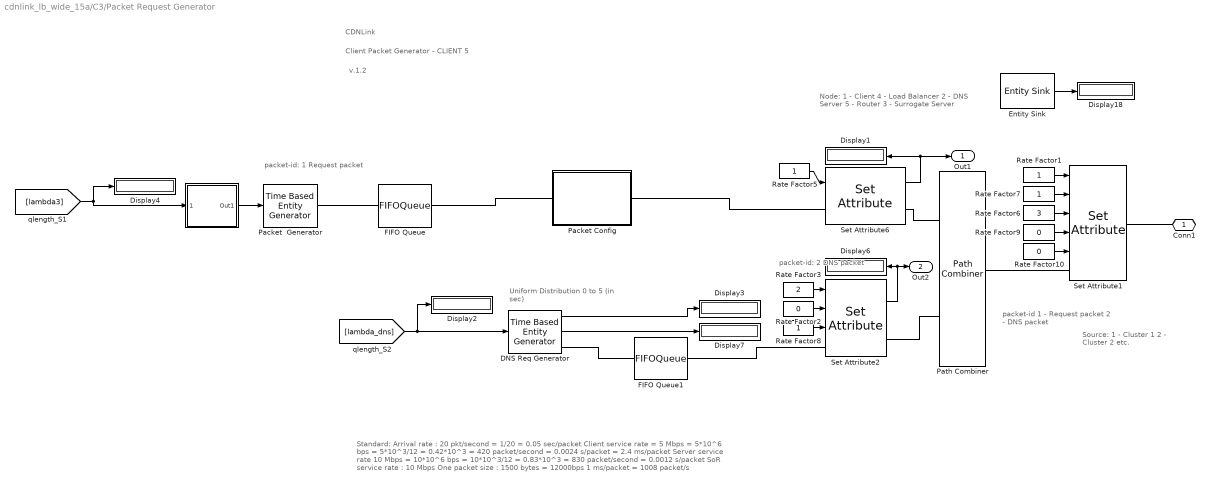
== system cdnlink_lb_wide_15a/C3/Packet Request Generator ==
  note: CDNLink
  note: Client Packet Generator - CLIENT 5
  note: Standard:
      | Arrival rate : 20 pkt/second = 1/20 = 0.05 sec/packet
      | Client service rate = 5 Mbps = 5*10^6 bps = 5*10^3/12 = 0.42*10^3 = 420 packet/second = 0.0024 s/packet = 2.4 ms/packet
      | Server service rate 10 Mbps = 10*10^6 bps = 10*10^3/12 = 0.83*10^3 = 830 packet/second = 0.0012 s/packet
      | SoR service rate : 10 Mbps
      | One packet size : 1500 bytes = 12000bps
      | 1 ms/packet = 1008 packet/s
  note: Node:
      | 1 - Client                     4 - Load Balancer
      | 2 - DNS Server            5 - Router
      | 3 - Surrogate Server
  note: packet-id
      | 1 - Request packet
      | 2 - DNS packet
  note: packet-id: 2
      | DNS packet
  note: Uniform Distribution
      | 0 to 5 (in sec)
  note: v.1.2
  note: Source:
      | 1 - Cluster 1
      | 2 - Cluster 2
      | etc.
  note: packet-id:  1
      | Request packet
  "  " : Subsystem  mask(Exponential Random Number Generator){seed=85274}
      mask prompts: seed "Initial seed"
      mask help: Output exponentially distributed random numbers with the input rate. Output is repeatable for a given seed.
      mask Display: disp('Exponential\n Distribution');
  DNS Req Generator : TimeBasedEntityGenerator  GenerateEntitiesUpon=Intergeneration time from port t  Distribution=Uniform  Period=10  InitialSeed=1715331  Maximum=5  Mean=0.05  ResponseWhenBlocked=Error  EntityType=Standard  StatNumberDeparted=on  StatAverageIntergenerationTime=on
      settings: OutputPortMap=o0,o2
  Display{1..4,6..7,18} (7 alike) : Display
  Entity Sink : EntitySink  StatNumberArrived=on
  FIFO Queue : FIFOQueue  Capacity=2000
  FIFO Queue1 : FIFOQueue  Capacity=2000
  Packet  Generator : TimeBasedEntityGenerator  GenerateEntitiesUpon=Intergeneration time from port t  Distribution=Exponential  Period=0.05  InitialSeed=1234  Mean=0.05  GenerateEntityAtSimulationStart=off  EntityType=Standard
  Packet Config : Subsystem
      mask Display: disp('Packet Config')
  Path Combiner : PathCombiner  NumberInputPorts=2
  Rate Factor{1,5,7..8} (4 alike) : Constant
  Rate Factor10 : Constant  Value=0
  Rate Factor2 : Constant  Value=0
  Rate Factor3 : Constant  Value=2
  Rate Factor6 : Constant  Value=3
  Rate Factor9 : Constant  Value=0
  Set Attribute1 : SetAttribute  AttributeName=node|reply|source|hop_count|router_id  AttributeFrom=Signal port|Signal port|Signal port|Signal port|Signal port  AttributeValue=1|1|1|1|1  AttributeTreatAsVector=1|1|1|1|1  EvaluatedAttributeValue={ [];[];[];[];[]}
      settings: InputPortMap=u0,u1,u2,u3,u4
  Set Attribute2 : SetAttribute  AttributeName=packet_id|content_time|dest  AttributeFrom=Signal port|Signal port|Signal port  AttributeValue=1|1|1  AttributeTreatAsVector=1|1|1  StatNumberDeparted=on  EvaluatedAttributeValue={ [];[];[]}
      settings: InputPortMap=u0,u1,u2
  Set Attribute6 : SetAttribute  AttributeName=packet_id  AttributeFrom=Signal port  StatNumberDeparted=on  EvaluatedAttributeValue={ []}
  Conn1 : PMIOPort  Port=1  Side=Right
  Out1 : Outport
  Out2 : Outport  Port=2
  wires:
  Rate Factor3/1 -> Set Attribute2/1
  Rate Factor8/1 -> Set Attribute2/3
  Rate Factor2/1 -> Set Attribute2/2
  Set Attribute2/1 -> Out2/1, Display6/1
  [lambda_dns] -> DNS Req Generator/1, Display2/1
  Set Attribute6/1 -> Display1/1, Out1/1
  Rate Factor5/1 -> Set Attribute6/1
  DNS Req Generator/2 -> Display7/1
  DNS Req Generator/1 -> Display3/1
  [lambda3] -> "  "/1(Arrival Rate), Display4/1
  "  "/1(Out1) -> Packet  Generator/1
  Entity Sink/1 -> Display18/1
  Rate Factor6/1 -> Set Attribute1/3
  Rate Factor7/1 -> Set Attribute1/2
  Rate Factor1/1 -> Set Attribute1/1
  Rate Factor9/1 -> Set Attribute1/4
  Rate Factor10/1 -> Set Attribute1/5
  connections:
  Path Combiner/RConn1 -- Set Attribute1/LConn1
  Path Combiner/LConn2 -- Set Attribute2/RConn1
  Path Combiner/LConn1 -- Set Attribute6/RConn1
  Packet Config/RConn1 -- Set Attribute6/LConn1
  FIFO Queue/LConn1 -- Packet  Generator/RConn1
  Packet Config/LConn1 -- FIFO Queue/RConn1
  FIFO Queue1/LConn1 -- DNS Req Generator/RConn1
  FIFO Queue1/RConn1 -- Set Attribute2/LConn1
  Conn1/RConn1 -- Set Attribute1/RConn1

== system cdnlink_lb_wide_15a/C3/Processing Module1 ==
  note: CDNLink
  note: Client Processing Module
  note: packet-id
      | 1 - Request packet
      | 2 - DNS packet
  note: Destination obtained from
      | DNS packet
  note: v.1.0
  AvgDelay SQ{1..2,4,6..9} (7 alike) : Display
  Display{1..3,5} (4 alike) : Display
  Entity Sink1 : EntitySink  StatNumberArrived=on
  Get Attribute : GetAttribute  AttributeName=packet_id|dest  AttributeMissing=Error|Error  AttributeDefaultValue=1|0  AttributeTreatAsVector=1|1  AttributeSendTiming=After entity departure|After entity departure  StatNumberDeparted=on  EvaluatedDefaultAttributeValue={ [];[]}
      settings: OutputPortMap=o0,o1,o2
  Get Attribute1 : GetAttribute  AttributeName=dest  AttributeDefaultValue=0  StatNumberDeparted=on  EvaluatedDefaultAttributeValue={ []}
      settings: OutputPortMap=o0,o1
  Output Switch : OutputSwitch  SwitchingCriterion=From attribute  AttributeName=packet_id  StatNumberDeparted=on
  Packet_id : OutputSwitch  NumberOutputPorts=2  SwitchingCriterion=From attribute  AttributeName=packet_id
  Packet_id1 : OutputSwitch  NumberOutputPorts=2  SwitchingCriterion=From attribute  AttributeName=packet_id
  Path Combiner : PathCombiner  NumberInputPorts=2
  Path Combiner1 : PathCombiner  NumberInputPorts=2  StatNumberDeparted=on
  Path Combiner2 : PathCombiner  NumberInputPorts=2  StatNumberDeparted=on
  Set Attribute14 : SetAttribute  AttributeName=dest  AttributeFrom=Signal port  AttributeValue=2  StatNumberDeparted=on  EvaluatedAttributeValue={ []}
  Start Timer : StartTimer  StatNumberDeparted=on
  From  Packet Generator : PMIOPort  Port=1  Side=Left
  To Router : PMIOPort  Port=2  Side=Right
  to sink : PMIOPort  Port=3  Side=Right
  From Router : PMIOPort  Port=4  Side=Left
  tag scope: dest_C3=global
  wires:
  Get Attribute1/1 -> AvgDelay SQ8/1
  Set Attribute14/1 -> AvgDelay SQ6/1
  Start Timer/1 -> AvgDelay SQ9/1
  Get Attribute1/2 -> [dest_C3], Set Attribute14/1, AvgDelay SQ7/1
  Path Combiner2/1 -> Display5/1
  Path Combiner1/1 -> Display1/1
  Get Attribute/3 -> AvgDelay SQ1/1
  Get Attribute/2 -> AvgDelay SQ2/1
  Entity Sink1/1 -> Display3/1
  Get Attribute/1 -> AvgDelay SQ4/1
  Output Switch/1 -> Display2/1
  connections:
  Output Switch/LConn1 -- Get Attribute/RConn1
  Path Combiner1/LConn2 -- Output Switch/RConn2
  Path Combiner1/RConn1 -- To Router/RConn1
  Path Combiner/RConn1 -- Get Attribute/LConn1
  Start Timer/RConn1 -- Path Combiner1/LConn1
  From  Packet Generator/RConn1 -- Packet_id/LConn1
  Packet_id/RConn2 -- Path Combiner/LConn2
  Packet_id/RConn1 -- Set Attribute14/LConn1
  Output Switch/RConn1 -- Start Timer/LConn1
  Set Attribute14/RConn1 -- Path Combiner/LConn1
  From Router/RConn1 -- Packet_id1/LConn1
  Packet_id1/RConn2 -- Get Attribute1/LConn1
  Get Attribute1/RConn1 -- Path Combiner2/LConn2
  Packet_id1/RConn1 -- Path Combiner2/LConn1
  Path Combiner2/RConn1 -- to sink/RConn1
  Output Switch/RConn3 -- Entity Sink1/LConn1

== system cdnlink_lb_wide_15a/C3/Sink1 ==
  note: Packet ID
      | 1 : Client request & Data
      | 2 : DNS request
  Display1 : Display
  Display2 : Display
  Display8 : Display
  Entity Sink : EntitySink  StatNumberArrived=on
  Entity Sink1 : EntitySink  StatNumberArrived=on
  "Output Switch: Packet ID " : OutputSwitch  NumberOutputPorts=2  SwitchingCriterion=From attribute  AttributeName=packet_id
  Read Timer : ReadTimer  TimerModeOption=Ignore  StatNumberDeparted=on  StatTimeElapsed=on  StatAverageTimeElapsed=on
      settings: OutputPortMap=o0,o2,o3
  Conn1 : PMIOPort  Port=1  Side=Left
  Out1 : Outport
  Out2 : Outport  Port=2
  tag scope: rtt_avg_c3=global, rtt_elaps_c3=global
  wires:
  Entity Sink/1 -> Out1/1, Display8/1
  Read Timer/1 -> Display1/1
  Entity Sink1/1 -> Out2/1, Display2/1
  Read Timer/2 -> [rtt_elaps_c3]
  Read Timer/3 -> [rtt_avg_c3]
  connections:
  Read Timer/RConn1 -- Entity Sink/LConn1
  Conn1/RConn1 -- "Output Switch: Packet ID "/LConn1
  "Output Switch: Packet ID "/RConn1 -- Read Timer/LConn1
  "Output Switch: Packet ID "/RConn2 -- Entity Sink1/LConn1

== system cdnlink_lb_wide_15a/R1/ 1 ==
  note: Exponential Distribution
      | Service Rate Generator
  note: CDNlink-NS
  note: 830 packet/ second = 10 Mbps
      | for Router --> 500 Mbps = 830*10*5 = 41500
      | for Server --> 100 Mbps = 830*10 = 8300
  "  " : Subsystem  mask(Exponential Random Number Generator){seed=85274}
      mask prompts: seed "Initial seed"
      mask help: Output exponentially distributed random numbers with the input rate. Output is repeatable for a given seed.
      mask Display: disp('Exponential\n Distribution');
  Display1 : Display
  Display4 : Display
  Service time : Outport
  wires:
  "  "/1(Out1) -> Display1/1, Service time/1
  [router3] -> Display4/1, "  "/1(Arrival Rate)
